simulink library "VSIGenLib"  (R2019b)
settings: Solver=VariableStepAuto  StartTime=0.0  StopTime=10.0  RelTol=1e-3
PostLoadFcn:
  | , if any(exist('dsrtsu_mdlpostloadfcn', 'file') ~= 0), dsrtsu_mdlpostloadfcn('Execute', bdroot); end,
undefined symbols (not defined in the file or in its folder): LIDAR, Ts_hil
libraries: simulink x76, $bdroot x46, etargetslib x30, ASCGenLib x26, dsmpblib x6
(part 2 of 3)

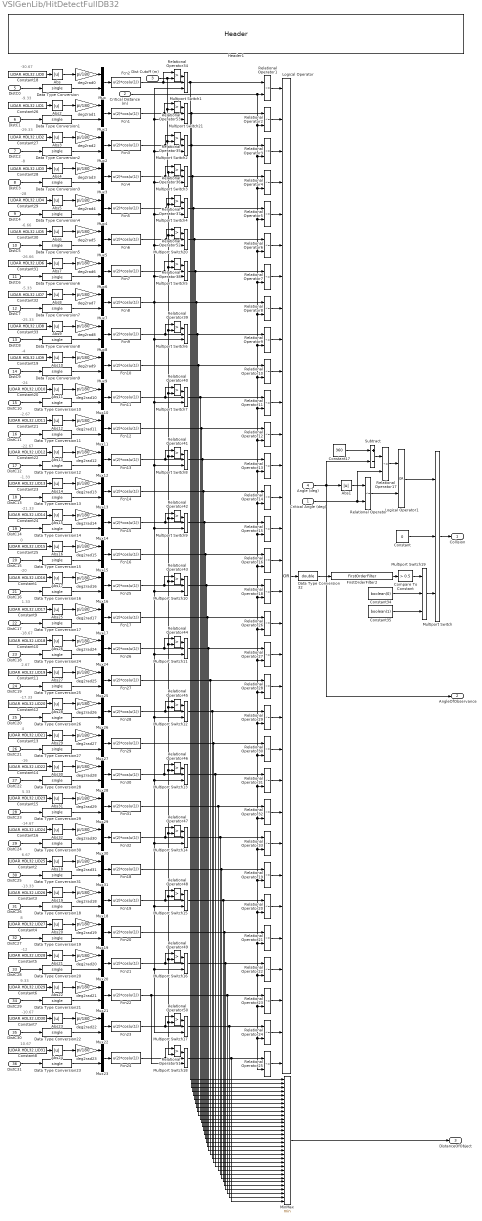
== system VSIGenLib/HitDetectFullDB32 ==
  note: -30.67
  note: -9.33
  note: -29.33
  note: -8
  note: -28
  note: -6.66
  note: -26.66
  note: -5.33
  note: -25.33
  note: -4
  note: -24
  note: -2.67
  note: 0
  note: -21.33
  note: -1.33
  note: -22.67
  note: -20
  note: 1.33
  note: -18.67
  note: 2.67
  note: -17.33
  note: 4
  note: -16
  note: 5.33
  note: -14.67
  note: 6.67
  note: -13.33
  note: 8
  note: 10.67
  note: -10.67
  note: 9.33
  note: -12
  Critical Angle (deg) : Inport
  Critical Distance (m) : Inport  Port=2
  Dist Cutoff (m) : Inport  Port=3
  Angle (deg) : Inport  Port=4
  DistC0 : Inport  Port=5
  DistC1 : Inport  Port=6
  DistC2 : Inport  Port=7
  DistC3 : Inport  Port=8
  DistC4 : Inport  Port=9
  DistC5 : Inport  Port=10
  DistC6 : Inport  Port=11
  DistC7 : Inport  Port=12
  DistC8 : Inport  Port=13
  DistC9 : Inport  Port=14
  DistC10 : Inport  Port=15
  DistC11 : Inport  Port=16
  DistC12 : Inport  Port=17
  DistC13 : Inport  Port=18
  DistC14 : Inport  Port=19
  DistC15 : Inport  Port=20
  DistC16 : Inport  Port=21
  DistC17 : Inport  Port=22
  DistC18 : Inport  Port=23
  DistC19 : Inport  Port=24
  DistC20 : Inport  Port=25
  DistC21 : Inport  Port=26
  DistC22 : Inport  Port=27
  DistC23 : Inport  Port=28
  DistC24 : Inport  Port=29
  DistC25 : Inport  Port=30
  DistC26 : Inport  Port=31
  DistC27 : Inport  Port=32
  DistC28 : Inport  Port=33
  DistC29 : Inport  Port=34
  DistC30 : Inport  Port=35
  DistC31 : Inport  Port=36
  Abs{,1..32} (33 alike) : Abs
  Compare To Constant : simulink/Logic and Bit Operations/Compare To Constant  relop=>  const=0.5  OutDataTypeStr=boolean
  Constant : Constant  Value=0
  Constant1 : Constant  Value=LIDAR.HDL32.LID16
  Constant10 : Constant  Value=LIDAR.HDL32.LID18
  Constant11 : Constant  Value=LIDAR.HDL32.LID19
  Constant12 : Constant  Value=LIDAR.HDL32.LID20
  Constant13 : Constant  Value=LIDAR.HDL32.LID21
  Constant14 : Constant  Value=LIDAR.HDL32.LID22
  Constant15 : Constant  Value=LIDAR.HDL32.LID23
  Constant16 : Constant  Value=LIDAR.HDL32.LID24
  Constant17 : Constant  Value=360
  Constant18 : Constant  Value=LIDAR.HDL32.LID0
  Constant19 : Constant  Value=LIDAR.HDL32.LID9
  Constant2 : Constant  Value=LIDAR.HDL32.LID25
  Constant20 : Constant  Value=LIDAR.HDL32.LID10
  Constant21 : Constant  Value=LIDAR.HDL32.LID11
  Constant22 : Constant  Value=LIDAR.HDL32.LID12
  Constant23 : Constant  Value=LIDAR.HDL32.LID13
  Constant24 : Constant  Value=LIDAR.HDL32.LID14
  Constant25 : Constant  Value=LIDAR.HDL32.LID15
  Constant26 : Constant  Value=LIDAR.HDL32.LID1
  Constant27 : Constant  Value=LIDAR.HDL32.LID2
  Constant28 : Constant  Value=LIDAR.HDL32.LID3
  Constant29 : Constant  Value=LIDAR.HDL32.LID4
  Constant3 : Constant  Value=LIDAR.HDL32.LID26
  Constant30 : Constant  Value=LIDAR.HDL32.LID5
  Constant31 : Constant  Value=LIDAR.HDL32.LID6
  Constant32 : Constant  Value=LIDAR.HDL32.LID7
  Constant33 : Constant  Value=LIDAR.HDL32.LID8
  Constant34 : Constant  Value=boolean(0)
  Constant35 : Constant  Value=boolean(1)
  Constant4 : Constant  Value=LIDAR.HDL32.LID27
  Constant5 : Constant  Value=LIDAR.HDL32.LID28
  Constant6 : Constant  Value=LIDAR.HDL32.LID29
  Constant7 : Constant  Value=LIDAR.HDL32.LID30
  Constant8 : Constant  Value=LIDAR.HDL32.LID31
  Constant9 : Constant  Value=LIDAR.HDL32.LID17
  Data Type Conversion{,1..31} (32 alike) : DataTypeConversion  OutDataTypeStr=single
  Data Type Conversion32 : DataTypeConversion  OutDataTypeStr=double
  Fcn{1..32} (32 alike) : Fcn  Expr=u(2)*cos(u(1))
  FirstOrderFilter2 : ASCGenLib/FirstOrderFilter  SystemSampleTime=-1
  Header1 : ASCGenLib/Header  not='L0 -30.67deg; L1 -9.33deg; L2 -29.33deg; L3 -8deg; L4 -28deg; L5 -6.66deg; L6 -26.66deg; L7 -5.33deg; L8 -25.33deg; L9 -4deg; L10 -24deg; L11 -2.67deg; L12 -22.67deg; L13 -1.33deg; L14 -21.33deg; L15 0deg\nL16 -20deg; L17 1.33deg; L18 -18.67deg; L19 2.67deg; L20 -17.33deg; L21 4deg; L22 -16deg; L23 5.33deg; L24 -14.67deg; L25 6.67deg; L26 -13.33deg; L27 8deg; L28 -12deg; L29 9.33deg; L30 -10.67deg; L31 10.67deg'
  Logical Operator : Logic  Operator=OR  Inputs=32  AllPortsSameDT=off  OutDataTypeStr=boolean
  Logical Operator1 : Logic  Operator=OR  AllPortsSameDT=off  OutDataTypeStr=boolean
  MinMax : MinMax  Inputs=32
  Multiport Switch{,1..21} (22 alike) : MultiPortSwitch  DataPortOrder=Zero-based contiguous  Inputs=2  zeroidx=on
  Mux{,1..31} (32 alike) : Mux  Inputs=2
  Relational Operator{,1..33} (34 alike) : RelationalOperator  Operator=<=  OutDataTypeStr=boolean  RndMeth=Simplest
  Relational Operator{34..53} (20 alike) : RelationalOperator  Operator=>  OutDataTypeStr=boolean  RndMeth=Simplest
  Subtract : Sum  Inputs=+-
  deg2rad{0..31} (32 alike) : Gain  Gain=pi/180  OutDataTypeStr=single
  Collision : Outport  VectorParamsAs1DForOutWhenUnconnected=off
  AngleOfObservance : Outport  Port=2  VectorParamsAs1DForOutWhenUnconnected=off
  DistanceOfObject : Outport  Port=3  VectorParamsAs1DForOutWhenUnconnected=off
  wires:
  Angle (deg)/1 -> Subtract/2, Abs1/1, AngleOfObservance/1
  Critical Angle (deg)/1 -> Relational Operator17/2, Relational Operator/2
  Relational Operator/1 -> Logical Operator1/2
  Constant/1 -> Multiport Switch/2
  Multiport Switch/1 -> Collision/1
  Relational Operator1/1 -> Logical Operator/1
  Constant18/1 -> Abs/1
  Mux/1 -> Fcn2/1
  Abs/1 -> deg2rad0/1
  Abs1/1 -> Relational Operator/1
  Constant26/1 -> Abs2/1
  Mux1/1 -> Fcn1/1
  Abs2/1 -> deg2rad1/1
  DistC0/1 -> Data Type Conversion/1
  DistC1/1 -> Data Type Conversion1/1
  Relational Operator2/1 -> Logical Operator/2
  Constant27/1 -> Abs3/1
  Mux2/1 -> Fcn3/1
  Abs3/1 -> deg2rad2/1
  Constant28/1 -> Abs4/1
  Mux3/1 -> Fcn4/1
  Abs4/1 -> deg2rad3/1
  DistC2/1 -> Data Type Conversion2/1
  DistC3/1 -> Data Type Conversion3/1
  Relational Operator3/1 -> Logical Operator/3
  Relational Operator4/1 -> Logical Operator/4
  Relational Operator5/1 -> Logical Operator/5
  Constant29/1 -> Abs5/1
  Abs5/1 -> deg2rad4/1
  Mux4/1 -> Fcn5/1
  deg2rad4/1 -> Mux4/1
  Constant30/1 -> Abs6/1
  Abs6/1 -> deg2rad5/1
  Mux5/1 -> Fcn6/1
  deg2rad5/1 -> Mux5/1
  DistC4/1 -> Data Type Conversion4/1
  DistC5/1 -> Data Type Conversion5/1
  Relational Operator6/1 -> Logical Operator/6
  Constant31/1 -> Abs7/1
  Abs7/1 -> deg2rad6/1
  Mux6/1 -> Fcn7/1
  deg2rad6/1 -> Mux6/1
  Constant32/1 -> Abs8/1
  Abs8/1 -> deg2rad7/1
  Mux7/1 -> Fcn8/1
  deg2rad7/1 -> Mux7/1
  DistC6/1 -> Data Type Conversion6/1
  DistC7/1 -> Data Type Conversion7/1
  Relational Operator7/1 -> Logical Operator/7
  Relational Operator8/1 -> Logical Operator/8
  Constant33/1 -> Abs9/1
  Abs9/1 -> deg2rad8/1
  Mux8/1 -> Fcn9/1
  deg2rad8/1 -> Mux8/1
  DistC8/1 -> Data Type Conversion8/1
  Relational Operator9/1 -> Logical Operator/9
  Relational Operator10/1 -> Logical Operator/10
  Constant19/1 -> Abs10/1
  Abs10/1 -> deg2rad9/1
  Mux9/1 -> Fcn10/1
  deg2rad9/1 -> Mux9/1
  Constant20/1 -> Abs11/1
  Abs11/1 -> deg2rad10/1
  Mux10/1 -> Fcn11/1
  deg2rad10/1 -> Mux10/1
  DistC9/1 -> Data Type Conversion9/1
  DistC10/1 -> Data Type Conversion10/1
  Relational Operator11/1 -> Logical Operator/11
  Constant21/1 -> Abs12/1
  Abs12/1 -> deg2rad11/1
  Mux11/1 -> Fcn12/1
  deg2rad11/1 -> Mux11/1
  Constant22/1 -> Abs13/1
  Abs13/1 -> deg2rad12/1
  Mux12/1 -> Fcn13/1
  deg2rad12/1 -> Mux12/1
  DistC11/1 -> Data Type Conversion11/1
  DistC12/1 -> Data Type Conversion12/1
  Relational Operator12/1 -> Logical Operator/12
  Relational Operator13/1 -> Logical Operator/13
  Constant23/1 -> Abs14/1
  Abs14/1 -> deg2rad13/1
  Mux13/1 -> Fcn14/1
  deg2rad13/1 -> Mux13/1
  Constant24/1 -> Abs15/1
  Abs15/1 -> deg2rad14/1
  Mux14/1 -> Fcn15/1
  deg2rad14/1 -> Mux14/1
  DistC13/1 -> Data Type Conversion13/1
  DistC14/1 -> Data Type Conversion14/1
  Relational Operator14/1 -> Logical Operator/14
  Relational Operator15/1 -> Logical Operator/15
  Constant25/1 -> Abs16/1
  Abs16/1 -> deg2rad15/1
  Mux15/1 -> Fcn16/1
  deg2rad15/1 -> Mux15/1
  DistC15/1 -> Data Type Conversion15/1
  Relational Operator16/1 -> Logical Operator/16
  Constant17/1 -> Subtract/1
  Subtract/1 -> Relational Operator17/1
  Logical Operator1/1 -> Multiport Switch/1
  Relational Operator17/1 -> Logical Operator1/1
  deg2rad0/1 -> Mux/1
  deg2rad1/1 -> Mux1/1
  deg2rad2/1 -> Mux2/1
  deg2rad3/1 -> Mux3/1
  MinMax/1 -> DistanceOfObject/1
  Data Type Conversion/1 -> Mux/2
  Data Type Conversion1/1 -> Mux1/2
  Data Type Conversion2/1 -> Mux2/2
  Data Type Conversion3/1 -> Mux3/2
  Data Type Conversion4/1 -> Mux4/2
  Data Type Conversion5/1 -> Mux5/2
  Data Type Conversion6/1 -> Mux6/2
  Data Type Conversion7/1 -> Mux7/2
  Data Type Conversion8/1 -> Mux8/2
  Data Type Conversion9/1 -> Mux9/2
  Data Type Conversion10/1 -> Mux10/2
  Data Type Conversion11/1 -> Mux11/2
  Data Type Conversion12/1 -> Mux12/2
  Data Type Conversion13/1 -> Mux13/2
  Data Type Conversion14/1 -> Mux14/2
  Data Type Conversion15/1 -> Mux15/2
  Constant1/1 -> Abs17/1
  Mux16/1 -> Fcn25/1
  Abs17/1 -> deg2rad16/1
  Constant9/1 -> Abs25/1
  Mux17/1 -> Fcn17/1
  Abs25/1 -> deg2rad17/1
  DistC16/1 -> Data Type Conversion16/1
  DistC17/1 -> Data Type Conversion17/1
  Constant10/1 -> Abs26/1
  Mux24/1 -> Fcn26/1
  Abs26/1 -> deg2rad24/1
  Constant11/1 -> Abs27/1
  Mux25/1 -> Fcn27/1
  Abs27/1 -> deg2rad25/1
  DistC18/1 -> Data Type Conversion24/1
  DistC19/1 -> Data Type Conversion25/1
  Constant12/1 -> Abs28/1
  Abs28/1 -> deg2rad26/1
  Mux26/1 -> Fcn28/1
  deg2rad26/1 -> Mux26/1
  Constant13/1 -> Abs29/1
  Abs29/1 -> deg2rad27/1
  Mux27/1 -> Fcn29/1
  deg2rad27/1 -> Mux27/1
  DistC20/1 -> Data Type Conversion26/1
  DistC21/1 -> Data Type Conversion27/1
  Constant14/1 -> Abs30/1
  Abs30/1 -> deg2rad28/1
  Mux28/1 -> Fcn30/1
  deg2rad28/1 -> Mux28/1
  Constant15/1 -> Abs31/1
  Abs31/1 -> deg2rad29/1
  Mux29/1 -> Fcn31/1
  deg2rad29/1 -> Mux29/1
  DistC22/1 -> Data Type Conversion28/1
  DistC23/1 -> Data Type Conversion29/1
  Constant16/1 -> Abs32/1
  Abs32/1 -> deg2rad30/1
  Mux30/1 -> Fcn32/1
  deg2rad30/1 -> Mux30/1
  DistC24/1 -> Data Type Conversion30/1
  Constant2/1 -> Abs18/1
  Abs18/1 -> deg2rad31/1
  Mux31/1 -> Fcn18/1
  deg2rad31/1 -> Mux31/1
  Constant3/1 -> Abs19/1
  Abs19/1 -> deg2rad18/1
  Mux18/1 -> Fcn19/1
  deg2rad18/1 -> Mux18/1
  DistC25/1 -> Data Type Conversion31/1
  DistC26/1 -> Data Type Conversion18/1
  Constant4/1 -> Abs20/1
  Abs20/1 -> deg2rad19/1
  Mux19/1 -> Fcn20/1
  deg2rad19/1 -> Mux19/1
  Constant5/1 -> Abs21/1
  Abs21/1 -> deg2rad20/1
  Mux20/1 -> Fcn21/1
  deg2rad20/1 -> Mux20/1
  DistC27/1 -> Data Type Conversion19/1
  DistC28/1 -> Data Type Conversion20/1
  Constant6/1 -> Abs22/1
  Abs22/1 -> deg2rad21/1
  Mux21/1 -> Fcn22/1
  deg2rad21/1 -> Mux21/1
  Constant7/1 -> Abs23/1
  Abs23/1 -> deg2rad22/1
  Mux22/1 -> Fcn23/1
  deg2rad22/1 -> Mux22/1
  DistC29/1 -> Data Type Conversion21/1
  DistC30/1 -> Data Type Conversion22/1
  Constant8/1 -> Abs24/1
  Abs24/1 -> deg2rad23/1
  Mux23/1 -> Fcn24/1
  deg2rad23/1 -> Mux23/1
  DistC31/1 -> Data Type Conversion23/1
  deg2rad16/1 -> Mux16/1
  deg2rad17/1 -> Mux17/1
  deg2rad24/1 -> Mux24/1
  deg2rad25/1 -> Mux25/1
  Data Type Conversion16/1 -> Mux16/2
  Data Type Conversion17/1 -> Mux17/2
  Data Type Conversion24/1 -> Mux24/2
  Data Type Conversion25/1 -> Mux25/2
  Data Type Conversion26/1 -> Mux26/2
  Data Type Conversion27/1 -> Mux27/2
  Data Type Conversion28/1 -> Mux28/2
  Data Type Conversion29/1 -> Mux29/2
  Data Type Conversion30/1 -> Mux30/2
  Data Type Conversion31/1 -> Mux31/2
  Data Type Conversion18/1 -> Mux18/2
  Data Type Conversion19/1 -> Mux19/2
  Data Type Conversion20/1 -> Mux20/2
  Data Type Conversion21/1 -> Mux21/2
  Data Type Conversion22/1 -> Mux22/2
  Data Type Conversion23/1 -> Mux23/2
  Relational Operator18/1 -> Logical Operator/17
  Relational Operator26/1 -> Logical Operator/18
  Relational Operator27/1 -> Logical Operator/19
  Relational Operator28/1 -> Logical Operator/20
  Relational Operator29/1 -> Logical Operator/21
  Relational Operator30/1 -> Logical Operator/22
  Relational Operator31/1 -> Logical Operator/23
  Relational Operator32/1 -> Logical Operator/24
  Relational Operator33/1 -> Logical Operator/25
  Relational Operator19/1 -> Logical Operator/26
  Relational Operator20/1 -> Logical Operator/27
  Relational Operator21/1 -> Logical Operator/28
  Relational Operator22/1 -> Logical Operator/29
  Relational Operator23/1 -> Logical Operator/30
  Relational Operator24/1 -> Logical Operator/31
  Relational Operator25/1 -> Logical Operator/32
  Critical Distance (m)/1 -> Relational Operator2/2, Relational Operator3/2, Relational Operator4/2, Relational Operator5/2, Relational Operator6/2, Relational Operator7/2, Relational Operator8/2, Relational Operator9/2, Relational Operator10/2, Relational Operator11/2, Relational Operator12/2, Relational Operator13/2, Relational Operator15/2, Relational Operator16/2, Relational Operator18/2, Relational Operator26/2, Relational Operator27/2, Relational Operator28/2, Relational Operator29/2, Relational Operator30/2, Relational Operator31/2, Relational Operator32/2, Relational Operator33/2, Relational Operator19/2, Relational Operator20/2, Relational Operator21/2, Relational Operator22/2, Relational Operator23/2, Relational Operator24/2, Relational Operator25/2, Relational Operator14/2, Relational Operator1/2
  Relational Operator34/1 -> Multiport Switch1/1
  Fcn2/1 -> Multiport Switch1/2, Relational Operator34/1
  Multiport Switch1/1 -> MinMax/1, Relational Operator1/1
  Relational Operator35/1 -> Multiport Switch2/1
  Multiport Switch2/1 -> MinMax/3, Relational Operator3/1
  Fcn3/1 -> Relational Operator35/1, Multiport Switch2/2
  Relational Operator36/1 -> Multiport Switch3/1
  Multiport Switch3/1 -> MinMax/4, Relational Operator4/1
  Fcn4/1 -> Multiport Switch3/2, Relational Operator36/1
  Relational Operator37/1 -> Multiport Switch4/1
  Fcn5/1 -> Relational Operator37/1, Multiport Switch4/2
  Multiport Switch4/1 -> MinMax/5, Relational Operator5/1
  Multiport Switch20/1 -> MinMax/6, Relational Operator6/1
  Relational Operator38/1 -> Multiport Switch5/1
  Multiport Switch5/1 -> MinMax/7, Relational Operator7/1
  Fcn7/1 -> Relational Operator38/1, Multiport Switch5/2
  Fcn8/1 -> MinMax/8, Relational Operator8/1, Multiport Switch6/3, Multiport Switch7/3, Multiport Switch10/3, Multiport Switch11/3, Multiport Switch12/3, Multiport Switch14/3, Multiport Switch15/3, Multiport Switch16/3, Multiport Switch17/3, Multiport Switch13/3, Multiport Switch9/3, Multiport Switch8/3, Multiport Switch5/3, Multiport Switch20/3, Multiport Switch4/3, Multiport Switch3/3, Multiport Switch21/3, Multiport Switch1/3, Multiport Switch2/3
  Relational Operator39/1 -> Multiport Switch6/1
  Fcn9/1 -> Relational Operator39/1, Multiport Switch6/2
  Multiport Switch6/1 -> MinMax/9, Relational Operator9/1
  Fcn10/1 -> MinMax/10, Relational Operator10/1
  Fcn11/1 -> Relational Operator40/1, Multiport Switch7/2
  Multiport Switch7/1 -> MinMax/11, Relational Operator11/1
  Fcn13/1 -> Relational Operator41/1, Multiport Switch8/2
  Multiport Switch8/1 -> MinMax/13, Relational Operator13/1
  Relational Operator40/1 -> Multiport Switch7/1
  Relational Operator41/1 -> Multiport Switch8/1
  Fcn14/1 -> MinMax/14, Relational Operator14/1
  Relational Operator42/1 -> Multiport Switch9/1
  Multiport Switch9/1 -> MinMax/15, Relational Operator15/1
  Fcn15/1 -> Relational Operator42/1, Multiport Switch9/2
  Fcn16/1 -> MinMax/16, Relational Operator16/1
  Relational Operator43/1 -> Multiport Switch10/1
  Fcn25/1 -> Relational Operator43/1, Multiport Switch10/2
  Multiport Switch10/1 -> MinMax/17, Relational Operator18/1
  Relational Operator44/1 -> Multiport Switch11/1
  Multiport Switch11/1 -> MinMax/19, Relational Operator27/1
  Fcn26/1 -> Relational Operator44/1, Multiport Switch11/2
  Fcn17/1 -> MinMax/18, Relational Operator26/1
  Fcn27/1 -> MinMax/20, Relational Operator28/1
  Relational Operator45/1 -> Multiport Switch12/1
  Multiport Switch12/1 -> MinMax/21, Relational Operator29/1
  Fcn28/1 -> Relational Operator45/1, Multiport Switch12/2
  Fcn29/1 -> MinMax/22, Relational Operator30/1
  Relational Operator46/1 -> Multiport Switch13/1
  Multiport Switch13/1 -> MinMax/23, Relational Operator31/1
  Fcn30/1 -> Relational Operator46/1, Multiport Switch13/2
  Relational Operator47/1 -> Multiport Switch14/1
  Multiport Switch14/1 -> MinMax/25, Relational Operator33/1
  Fcn32/1 -> Relational Operator47/1, Multiport Switch14/2
  Fcn31/1 -> MinMax/24, Relational Operator32/1
  Fcn18/1 -> MinMax/26, Relational Operator19/1
  Relational Operator48/1 -> Multiport Switch15/1
  Multiport Switch15/1 -> MinMax/27, Relational Operator20/1
  Fcn19/1 -> Relational Operator48/1, Multiport Switch15/2
  Fcn20/1 -> MinMax/28, Relational Operator21/1
  Relational Operator49/1 -> Multiport Switch16/1
  Multiport Switch16/1 -> MinMax/29, Relational Operator22/1
  Fcn21/1 -> Relational Operator49/1, Multiport Switch16/2
  Relational Operator50/1 -> Multiport Switch17/1
  Multiport Switch17/1 -> MinMax/31, Relational Operator24/1
  Fcn23/1 -> Relational Operator50/1, Multiport Switch17/2
  Fcn12/1 -> MinMax/12, Relational Operator12/1
  Fcn22/1 -> Multiport Switch18/3, MinMax/30, Relational Operator23/1
  Relational Operator51/1 -> Multiport Switch18/1
  Multiport Switch18/1 -> MinMax/32, Relational Operator25/1
  Fcn24/1 -> Relational Operator51/1, Multiport Switch18/2
  FirstOrderFilter2/1 -> Compare To Constant/1
  Constant34/1 -> Multiport Switch19/2
  Constant35/1 -> Multiport Switch19/3
  Compare To Constant/1 -> Multiport Switch19/1
  Multiport Switch19/1 -> Multiport Switch/3
  Data Type Conversion32/1 -> FirstOrderFilter2/1
  Logical Operator/1 -> Data Type Conversion32/1
  Relational Operator52/1 -> Multiport Switch20/1
  Fcn6/1 -> Relational Operator52/1, Multiport Switch20/2
  Fcn1/1 -> Relational Operator53/1, Multiport Switch21/2
  Relational Operator53/1 -> Multiport Switch21/1
  Dist Cutoff (m)/1 -> Relational Operator53/2, Relational Operator52/2, Relational Operator47/2, Relational Operator48/2, Relational Operator49/2, Relational Operator51/2, Relational Operator50/2, Relational Operator46/2, Relational Operator45/2, Relational Operator44/2, Relational Operator43/2, Relational Operator42/2, Relational Operator41/2, Relational Operator40/2, Relational Operator39/2, Relational Operator38/2, Relational Operator37/2, Relational Operator36/2, Relational Operator35/2, Relational Operator34/2
  Multiport Switch21/1 -> MinMax/2, Relational Operator2/1

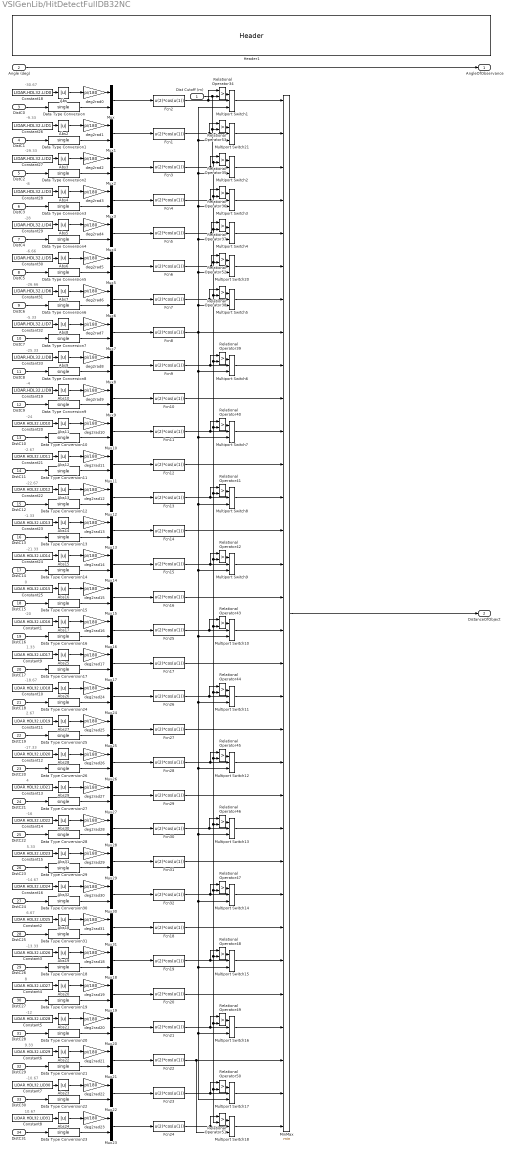
== system VSIGenLib/HitDetectFullDB32NC ==
  note: -30.67
  note: -9.33
  note: -8
  note: -6.66
  note: -26.66
  note: -5.33
  note: -4
  note: -24
  note: -2.67
  note: 0
  note: -1.33
  note: -22.67
  note: -29.33
  note: -20
  note: 1.33
  note: -28
  note: -18.67
  note: 2.67
  note: -17.33
  note: 4
  note: -25.33
  note: -16
  note: -14.67
  note: -13.33
  note: -21.33
  note: 8
  note: 10.67
  note: -10.67
  note: 9.33
  note: 5.33
  note: -12
  note: 6.67
  Dist Cutoff (m) : Inport
  Angle (deg) : Inport  Port=2
  DistC0 : Inport  Port=3
  DistC1 : Inport  Port=4
  DistC2 : Inport  Port=5
  DistC3 : Inport  Port=6
  DistC4 : Inport  Port=7
  DistC5 : Inport  Port=8
  DistC6 : Inport  Port=9
  DistC7 : Inport  Port=10
  DistC8 : Inport  Port=11
  DistC9 : Inport  Port=12
  DistC10 : Inport  Port=13
  DistC11 : Inport  Port=14
  DistC12 : Inport  Port=15
  DistC13 : Inport  Port=16
  DistC14 : Inport  Port=17
  DistC15 : Inport  Port=18
  DistC16 : Inport  Port=19
  DistC17 : Inport  Port=20
  DistC18 : Inport  Port=21
  DistC19 : Inport  Port=22
  DistC20 : Inport  Port=23
  DistC21 : Inport  Port=24
  DistC22 : Inport  Port=25
  DistC23 : Inport  Port=26
  DistC24 : Inport  Port=27
  DistC25 : Inport  Port=28
  DistC26 : Inport  Port=29
  DistC27 : Inport  Port=30
  DistC28 : Inport  Port=31
  DistC29 : Inport  Port=32
  DistC30 : Inport  Port=33
  DistC31 : Inport  Port=34
  Abs{,2..32} (32 alike) : Abs
  Constant1 : Constant  Value=LIDAR.HDL32.LID16
  Constant10 : Constant  Value=LIDAR.HDL32.LID18
  Constant11 : Constant  Value=LIDAR.HDL32.LID19
  Constant12 : Constant  Value=LIDAR.HDL32.LID20
  Constant13 : Constant  Value=LIDAR.HDL32.LID21
  Constant14 : Constant  Value=LIDAR.HDL32.LID22
  Constant15 : Constant  Value=LIDAR.HDL32.LID23
  Constant16 : Constant  Value=LIDAR.HDL32.LID24
  Constant18 : Constant  Value=LIDAR.HDL32.LID0
  Constant19 : Constant  Value=LIDAR.HDL32.LID9
  Constant2 : Constant  Value=LIDAR.HDL32.LID25
  Constant20 : Constant  Value=LIDAR.HDL32.LID10
  Constant21 : Constant  Value=LIDAR.HDL32.LID11
  Constant22 : Constant  Value=LIDAR.HDL32.LID12
  Constant23 : Constant  Value=LIDAR.HDL32.LID13
  Constant24 : Constant  Value=LIDAR.HDL32.LID14
  Constant25 : Constant  Value=LIDAR.HDL32.LID15
  Constant26 : Constant  Value=LIDAR.HDL32.LID1
  Constant27 : Constant  Value=LIDAR.HDL32.LID2
  Constant28 : Constant  Value=LIDAR.HDL32.LID3
  Constant29 : Constant  Value=LIDAR.HDL32.LID4
  Constant3 : Constant  Value=LIDAR.HDL32.LID26
  Constant30 : Constant  Value=LIDAR.HDL32.LID5
  Constant31 : Constant  Value=LIDAR.HDL32.LID6
  Constant32 : Constant  Value=LIDAR.HDL32.LID7
  Constant33 : Constant  Value=LIDAR.HDL32.LID8
  Constant4 : Constant  Value=LIDAR.HDL32.LID27
  Constant5 : Constant  Value=LIDAR.HDL32.LID28
  Constant6 : Constant  Value=LIDAR.HDL32.LID29
  Constant7 : Constant  Value=LIDAR.HDL32.LID30
  Constant8 : Constant  Value=LIDAR.HDL32.LID31
  Constant9 : Constant  Value=LIDAR.HDL32.LID17
  Data Type Conversion{,1..31} (32 alike) : DataTypeConversion  OutDataTypeStr=single
  Fcn{1..32} (32 alike) : Fcn  Expr=u(2)*cos(u(1))
  Header1 : ASCGenLib/Header  not='L0 -30.67deg; L1 -9.33deg; L2 -29.33deg; L3 -8deg; L4 -28deg; L5 -6.66deg; L6 -26.66deg; L7 -5.33deg; L8 -25.33deg; L9 -4deg; L10 -24deg; L11 -2.67deg; L12 -22.67deg; L13 -1.33deg; L14 -21.33deg; L15 0deg\nL16 -20deg; L17 1.33deg; L18 -18.67deg; L19 2.67deg; L20 -17.33deg; L21 4deg; L22 -16deg; L23 5.33deg; L24 -14.67deg; L25 6.67deg; L26 -13.33deg; L27 8deg; L28 -12deg; L29 9.33deg; L30 -10.67deg; L31 10.67deg'
  MinMax : MinMax  Inputs=32
  Multiport Switch{1..18,20..21} (20 alike) : MultiPortSwitch  DataPortOrder=Zero-based contiguous  Inputs=2  zeroidx=on
  Mux{,1..31} (32 alike) : Mux  Inputs=2
  Relational Operator{34..53} (20 alike) : RelationalOperator  Operator=>  OutDataTypeStr=boolean  RndMeth=Simplest
  deg2rad{0..31} (32 alike) : Gain  Gain=pi/180  OutDataTypeStr=single
  AngleOfObservance : Outport  VectorParamsAs1DForOutWhenUnconnected=off
  DistanceOfObject : Outport  Port=2  VectorParamsAs1DForOutWhenUnconnected=off
  wires:
  Multiport Switch16/1 -> MinMax/29
  Mux14/1 -> Fcn15/1
  Multiport Switch18/1 -> MinMax/32
  Mux17/1 -> Fcn17/1
  Abs6/1 -> deg2rad5/1
  Constant6/1 -> Abs22/1
  DistC3/1 -> Data Type Conversion3/1
  Relational Operator46/1 -> Multiport Switch13/1
  Dist Cutoff (m)/1 -> Relational Operator53/2, Relational Operator52/2, Relational Operator47/2, Relational Operator48/2, Relational Operator49/2, Relational Operator51/2, Relational Operator50/2, Relational Operator46/2, Relational Operator45/2, Relational Operator44/2, Relational Operator43/2, Relational Operator42/2, Relational Operator41/2, Relational Operator40/2, Relational Operator39/2, Relational Operator38/2, Relational Operator37/2, Relational Operator36/2, Relational Operator35/2, Relational Operator34/2
  deg2rad23/1 -> Mux23/1
  Multiport Switch14/1 -> MinMax/25
  Fcn2/1 -> Multiport Switch1/2, Relational Operator34/1
  Relational Operator40/1 -> Multiport Switch7/1
  Data Type Conversion/1 -> Mux/2
  DistC9/1 -> Data Type Conversion9/1
  DistC24/1 -> Data Type Conversion30/1
  Mux9/1 -> Fcn10/1
  deg2rad19/1 -> Mux19/1
  DistC5/1 -> Data Type Conversion5/1
  DistC0/1 -> Data Type Conversion/1
  Multiport Switch17/1 -> MinMax/31
  DistC25/1 -> Data Type Conversion31/1
  Fcn6/1 -> Relational Operator52/1, Multiport Switch20/2
  Abs24/1 -> deg2rad23/1
  Constant27/1 -> Abs3/1
  Constant8/1 -> Abs24/1
  Fcn21/1 -> Relational Operator49/1, Multiport Switch16/2
  Abs31/1 -> deg2rad29/1
  Multiport Switch8/1 -> MinMax/13
  DistC10/1 -> Data Type Conversion10/1
  deg2rad11/1 -> Mux11/1
  Relational Operator49/1 -> Multiport Switch16/1
  DistC27/1 -> Data Type Conversion19/1
  Abs15/1 -> deg2rad14/1
  Multiport Switch13/1 -> MinMax/23
  Relational Operator41/1 -> Multiport Switch8/1
  Fcn16/1 -> MinMax/16
  Fcn1/1 -> Relational Operator53/1, Multiport Switch21/2
  Fcn19/1 -> Relational Operator48/1, Multiport Switch15/2
  Data Type Conversion21/1 -> Mux21/2
  Fcn27/1 -> MinMax/20
  Fcn30/1 -> Relational Operator46/1, Multiport Switch13/2
  Multiport Switch20/1 -> MinMax/6
  Relational Operator39/1 -> Multiport Switch6/1
  DistC8/1 -> Data Type Conversion8/1
  Abs25/1 -> deg2rad17/1
  Mux20/1 -> Fcn21/1
  Abs/1 -> deg2rad0/1
  Data Type Conversion24/1 -> Mux24/2
  deg2rad12/1 -> Mux12/1
  Constant5/1 -> Abs21/1
  Fcn26/1 -> Relational Operator44/1, Multiport Switch11/2
  Fcn20/1 -> MinMax/28
  Relational Operator53/1 -> Multiport Switch21/1
  Fcn24/1 -> Relational Operator51/1, Multiport Switch18/2
  Fcn13/1 -> Relational Operator41/1, Multiport Switch8/2
  Fcn23/1 -> Relational Operator50/1, Multiport Switch17/2
  Relational Operator43/1 -> Multiport Switch10/1
  deg2rad16/1 -> Mux16/1
  Abs10/1 -> deg2rad9/1
  Relational Operator50/1 -> Multiport Switch17/1
  Abs22/1 -> deg2rad21/1
  deg2rad18/1 -> Mux18/1
  Multiport Switch9/1 -> MinMax/15
  Multiport Switch3/1 -> MinMax/4
  Mux23/1 -> Fcn24/1
  Fcn14/1 -> MinMax/14
  DistC11/1 -> Data Type Conversion11/1
  Constant13/1 -> Abs29/1
  Fcn10/1 -> MinMax/10
  Relational Operator38/1 -> Multiport Switch5/1
  Data Type Conversion1/1 -> Mux1/2
  Fcn9/1 -> Relational Operator39/1, Multiport Switch6/2
  Fcn8/1 -> MinMax/8, Multiport Switch6/3, Multiport Switch7/3, Multiport Switch10/3, Multiport Switch11/3, Multiport Switch12/3, Multiport Switch14/3, Multiport Switch15/3, Multiport Switch16/3, Multiport Switch17/3, Multiport Switch13/3, Multiport Switch9/3, Multiport Switch8/3, Multiport Switch5/3, Multiport Switch20/3, Multiport Switch4/3, Multiport Switch3/3, Multiport Switch21/3, Multiport Switch1/3, Multiport Switch2/3
  Constant9/1 -> Abs25/1
  Fcn12/1 -> MinMax/12
  Relational Operator48/1 -> Multiport Switch15/1
  Relational Operator52/1 -> Multiport Switch20/1
  Fcn28/1 -> Relational Operator45/1, Multiport Switch12/2
  Relational Operator37/1 -> Multiport Switch4/1
  deg2rad10/1 -> Mux10/1
  DistC26/1 -> Data Type Conversion18/1
  Multiport Switch10/1 -> MinMax/17
  deg2rad3/1 -> Mux3/1
  Multiport Switch5/1 -> MinMax/7
  Relational Operator44/1 -> Multiport Switch11/1
  Multiport Switch4/1 -> MinMax/5
  Fcn17/1 -> MinMax/18
  Fcn32/1 -> Relational Operator47/1, Multiport Switch14/2
  Fcn4/1 -> Multiport Switch3/2, Relational Operator36/1
  Relational Operator34/1 -> Multiport Switch1/1
  Abs23/1 -> deg2rad22/1
  Relational Operator36/1 -> Multiport Switch3/1
  Fcn3/1 -> Relational Operator35/1, Multiport Switch2/2
  Relational Operator35/1 -> Multiport Switch2/1
  deg2rad0/1 -> Mux/1
  Multiport Switch1/1 -> MinMax/1
  Data Type Conversion29/1 -> Mux29/2
  Data Type Conversion9/1 -> Mux9/2
  Data Type Conversion7/1 -> Mux7/2
  Fcn5/1 -> Relational Operator37/1, Multiport Switch4/2
  Constant3/1 -> Abs19/1
  deg2rad22/1 -> Mux22/1
  Abs32/1 -> deg2rad30/1
  DistC12/1 -> Data Type Conversion12/1
  Data Type Conversion26/1 -> Mux26/2
  Constant23/1 -> Abs14/1
  Data Type Conversion22/1 -> Mux22/2
  Mux27/1 -> Fcn29/1
  Data Type Conversion20/1 -> Mux20/2
  Data Type Conversion19/1 -> Mux19/2
  Mux19/1 -> Fcn20/1
  Data Type Conversion30/1 -> Mux30/2
  Data Type Conversion28/1 -> Mux28/2
  Data Type Conversion27/1 -> Mux27/2
  Relational Operator47/1 -> Multiport Switch14/1
  DistC17/1 -> Data Type Conversion17/1
  Data Type Conversion6/1 -> Mux6/2
  Constant10/1 -> Abs26/1
  Data Type Conversion16/1 -> Mux16/2
  Abs9/1 -> deg2rad8/1
  Fcn25/1 -> Relational Operator43/1, Multiport Switch10/2
  deg2rad24/1 -> Mux24/1
  deg2rad17/1 -> Mux17/1
  DistC31/1 -> Data Type Conversion23/1
  DistC30/1 -> Data Type Conversion22/1
  Constant11/1 -> Abs27/1
  Mux21/1 -> Fcn22/1
  Constant16/1 -> Abs32/1
  DistC28/1 -> Data Type Conversion20/1
  deg2rad20/1 -> Mux20/1
  Data Type Conversion3/1 -> Mux3/2
  deg2rad21/1 -> Mux21/1
  Abs21/1 -> deg2rad20/1
  Abs20/1 -> deg2rad19/1
  Constant4/1 -> Abs20/1
  deg2rad2/1 -> Mux2/1
  Abs19/1 -> deg2rad18/1
  deg2rad14/1 -> Mux14/1
  Abs18/1 -> deg2rad31/1
  Mux31/1 -> Fcn18/1
  Constant2/1 -> Abs18/1
  Abs26/1 -> deg2rad24/1
  deg2rad30/1 -> Mux30/1
  Mux30/1 -> Fcn32/1
  Constant15/1 -> Abs31/1
  Data Type Conversion17/1 -> Mux17/2
  Abs14/1 -> deg2rad13/1
  Fcn15/1 -> Relational Operator42/1, Multiport Switch9/2
  DistC16/1 -> Data Type Conversion16/1
  Constant18/1 -> Abs/1
  DistC21/1 -> Data Type Conversion27/1
  DistC20/1 -> Data Type Conversion26/1
  Mux25/1 -> Fcn27/1
  deg2rad27/1 -> Mux27/1
  deg2rad26/1 -> Mux26/1
  Multiport Switch12/1 -> MinMax/21
  Mux26/1 -> Fcn28/1
  Abs28/1 -> deg2rad26/1
  Constant12/1 -> Abs28/1
  Multiport Switch21/1 -> MinMax/2
  Mux12/1 -> Fcn13/1
  Abs27/1 -> deg2rad25/1
  Mux24/1 -> Fcn26/1
  Relational Operator42/1 -> Multiport Switch9/1
  Fcn11/1 -> Relational Operator40/1, Multiport Switch7/2
  deg2rad9/1 -> Mux9/1
  Abs17/1 -> deg2rad16/1
  Constant7/1 -> Abs23/1
  Mux16/1 -> Fcn25/1
  Constant1/1 -> Abs17/1
  deg2rad29/1 -> Mux29/1
  Data Type Conversion15/1 -> Mux15/2
  Multiport Switch6/1 -> MinMax/9
  Mux/1 -> Fcn2/1
  Data Type Conversion14/1 -> Mux14/2
  Data Type Conversion13/1 -> Mux13/2
  Mux18/1 -> Fcn19/1
  Data Type Conversion12/1 -> Mux12/2
  Data Type Conversion10/1 -> Mux10/2
  Data Type Conversion23/1 -> Mux23/2
  Data Type Conversion8/1 -> Mux8/2
  Data Type Conversion25/1 -> Mux25/2
  Abs29/1 -> deg2rad27/1
  Data Type Conversion5/1 -> Mux5/2
  DistC22/1 -> Data Type Conversion28/1
  Fcn7/1 -> Relational Operator38/1, Multiport Switch5/2
  Multiport Switch2/1 -> MinMax/3
  Data Type Conversion4/1 -> Mux4/2
  Abs11/1 -> deg2rad10/1
  DistC13/1 -> Data Type Conversion13/1
  deg2rad31/1 -> Mux31/1
  Abs13/1 -> deg2rad12/1
  Abs12/1 -> deg2rad11/1
  Constant22/1 -> Abs13/1
  Constant20/1 -> Abs11/1
  Mux28/1 -> Fcn30/1
  Abs16/1 -> deg2rad15/1
  Relational Operator51/1 -> Multiport Switch18/1
  Constant19/1 -> Abs10/1
  Constant24/1 -> Abs15/1
  Multiport Switch15/1 -> MinMax/27
  deg2rad8/1 -> Mux8/1
  deg2rad15/1 -> Mux15/1
  Mux22/1 -> Fcn23/1
  Mux29/1 -> Fcn31/1
  Mux8/1 -> Fcn9/1
  Data Type Conversion18/1 -> Mux18/2
  Constant26/1 -> Abs2/1
  Fcn18/1 -> MinMax/26
  DistC6/1 -> Data Type Conversion6/1
  Abs8/1 -> deg2rad7/1
  DistC23/1 -> Data Type Conversion29/1
  Constant32/1 -> Abs8/1
  deg2rad1/1 -> Mux1/1
  Data Type Conversion11/1 -> Mux11/2
  deg2rad6/1 -> Mux6/1
  Fcn31/1 -> MinMax/24
  DistC14/1 -> Data Type Conversion14/1
  deg2rad25/1 -> Mux25/1
  Constant31/1 -> Abs7/1
  DistC4/1 -> Data Type Conversion4/1
  deg2rad5/1 -> Mux5/1
  Data Type Conversion2/1 -> Mux2/2
  Data Type Conversion31/1 -> Mux31/2
  Mux5/1 -> Fcn6/1
  Constant30/1 -> Abs6/1
  deg2rad28/1 -> Mux28/1
  deg2rad4/1 -> Mux4/1
  Fcn22/1 -> MinMax/30, Multiport Switch18/3
  Multiport Switch11/1 -> MinMax/19
  Abs5/1 -> deg2rad4/1
  DistC18/1 -> Data Type Conversion24/1
  Mux11/1 -> Fcn12/1
  DistC29/1 -> Data Type Conversion21/1
  Constant29/1 -> Abs5/1
  deg2rad13/1 -> Mux13/1
  DistC15/1 -> Data Type Conversion15/1
  DistC1/1 -> Data Type Conversion1/1
  Mux7/1 -> Fcn8/1
  Mux1/1 -> Fcn1/1
  deg2rad7/1 -> Mux7/1
  DistC7/1 -> Data Type Conversion7/1
  DistC19/1 -> Data Type Conversion25/1
  Constant25/1 -> Abs16/1
  Abs4/1 -> deg2rad3/1
  Constant28/1 -> Abs4/1
  Abs7/1 -> deg2rad6/1
  Abs3/1 -> deg2rad2/1
  Constant33/1 -> Abs9/1
  Abs30/1 -> deg2rad28/1
  Mux2/1 -> Fcn3/1
  Fcn29/1 -> MinMax/22
  Mux10/1 -> Fcn11/1
  Abs2/1 -> deg2rad1/1
  Mux13/1 -> Fcn14/1
  Mux15/1 -> Fcn16/1
  Mux4/1 -> Fcn5/1
  Angle (deg)/1 -> AngleOfObservance/1
  Constant21/1 -> Abs12/1
  Relational Operator45/1 -> Multiport Switch12/1
  Mux3/1 -> Fcn4/1
  Constant14/1 -> Abs30/1
  Mux6/1 -> Fcn7/1
  Multiport Switch7/1 -> MinMax/11
  DistC2/1 -> Data Type Conversion2/1
  MinMax/1 -> DistanceOfObject/1

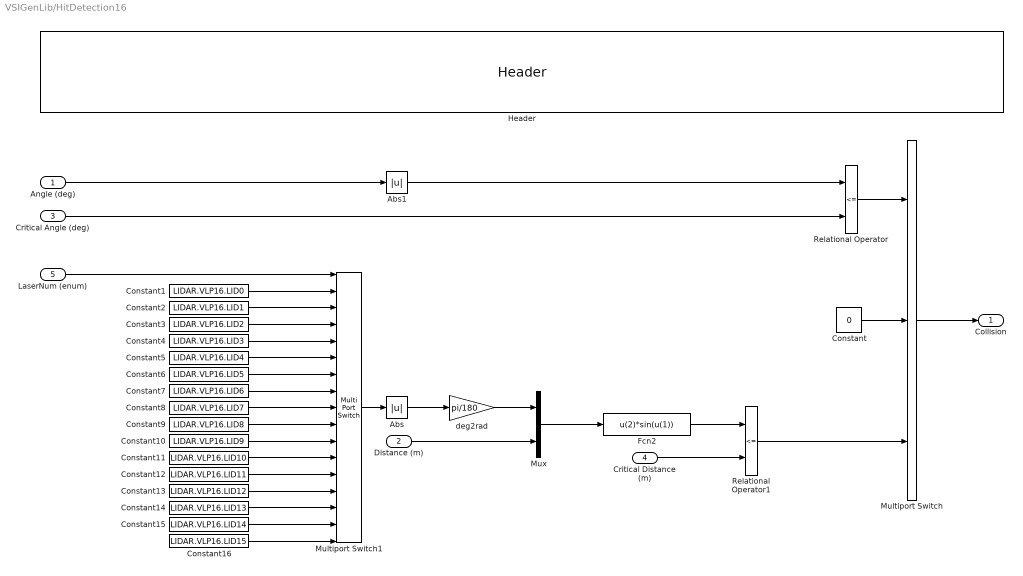
== system VSIGenLib/HitDetection16 ==
  Angle (deg) : Inport
  Distance (m) : Inport  Port=2
  Critical Angle (deg) : Inport  Port=3
  Critical Distance (m) : Inport  Port=4
  LaserNum (enum) : Inport  Port=5
  Abs : Abs
  Abs1 : Abs
  Constant : Constant  Value=0
  Constant1 : Constant  Value=LIDAR.VLP16.LID0
  Constant10 : Constant  Value=LIDAR.VLP16.LID9
  Constant11 : Constant  Value=LIDAR.VLP16.LID10
  Constant12 : Constant  Value=LIDAR.VLP16.LID11
  Constant13 : Constant  Value=LIDAR.VLP16.LID12
  Constant14 : Constant  Value=LIDAR.VLP16.LID13
  Constant15 : Constant  Value=LIDAR.VLP16.LID14
  Constant16 : Constant  Value=LIDAR.VLP16.LID15
  Constant2 : Constant  Value=LIDAR.VLP16.LID1
  Constant3 : Constant  Value=LIDAR.VLP16.LID2
  Constant4 : Constant  Value=LIDAR.VLP16.LID3
  Constant5 : Constant  Value=LIDAR.VLP16.LID4
  Constant6 : Constant  Value=LIDAR.VLP16.LID5
  Constant7 : Constant  Value=LIDAR.VLP16.LID6
  Constant8 : Constant  Value=LIDAR.VLP16.LID7
  Constant9 : Constant  Value=LIDAR.VLP16.LID8
  Fcn2 : Fcn  Expr=u(2)*sin(u(1))
  Header : $bdroot/Header  not=''
  Multiport Switch : MultiPortSwitch  DataPortOrder=Zero-based contiguous  Inputs=2  zeroidx=on
  Multiport Switch1 : MultiPortSwitch  DataPortOrder=Zero-based contiguous  Inputs=16  zeroidx=on
  Mux : Mux  Inputs=2
  Relational Operator : RelationalOperator  Operator=<=  OutDataTypeStr=boolean  RndMeth=Simplest
  Relational Operator1 : RelationalOperator  Operator=<=  OutDataTypeStr=boolean  RndMeth=Simplest
  deg2rad : Gain  Gain=pi/180
  Collision : Outport  VectorParamsAs1DForOutWhenUnconnected=off
  wires:
  Angle (deg)/1 -> Abs1/1
  Critical Angle (deg)/1 -> Relational Operator/2
  Distance (m)/1 -> Mux/2
  Critical Distance (m)/1 -> Relational Operator1/2
  Relational Operator/1 -> Multiport Switch/1
  Constant/1 -> Multiport Switch/2
  Multiport Switch/1 -> Collision/1
  Relational Operator1/1 -> Multiport Switch/3
  LaserNum (enum)/1 -> Multiport Switch1/1
  Constant1/1 -> Multiport Switch1/2
  Constant2/1 -> Multiport Switch1/3
  Constant9/1 -> Multiport Switch1/10
  Constant10/1 -> Multiport Switch1/11
  Constant7/1 -> Multiport Switch1/8
  Constant8/1 -> Multiport Switch1/9
  Constant3/1 -> Multiport Switch1/4
  Constant4/1 -> Multiport Switch1/5
  Constant15/1 -> Multiport Switch1/16
  Constant16/1 -> Multiport Switch1/17
  Constant5/1 -> Multiport Switch1/6
  Constant6/1 -> Multiport Switch1/7
  Constant13/1 -> Multiport Switch1/14
  Constant14/1 -> Multiport Switch1/15
  Constant11/1 -> Multiport Switch1/12
  Constant12/1 -> Multiport Switch1/13
  Multiport Switch1/1 -> Abs/1
  Abs/1 -> deg2rad/1
  Mux/1 -> Fcn2/1
  deg2rad/1 -> Mux/1
  Fcn2/1 -> Relational Operator1/1
  Abs1/1 -> Relational Operator/1

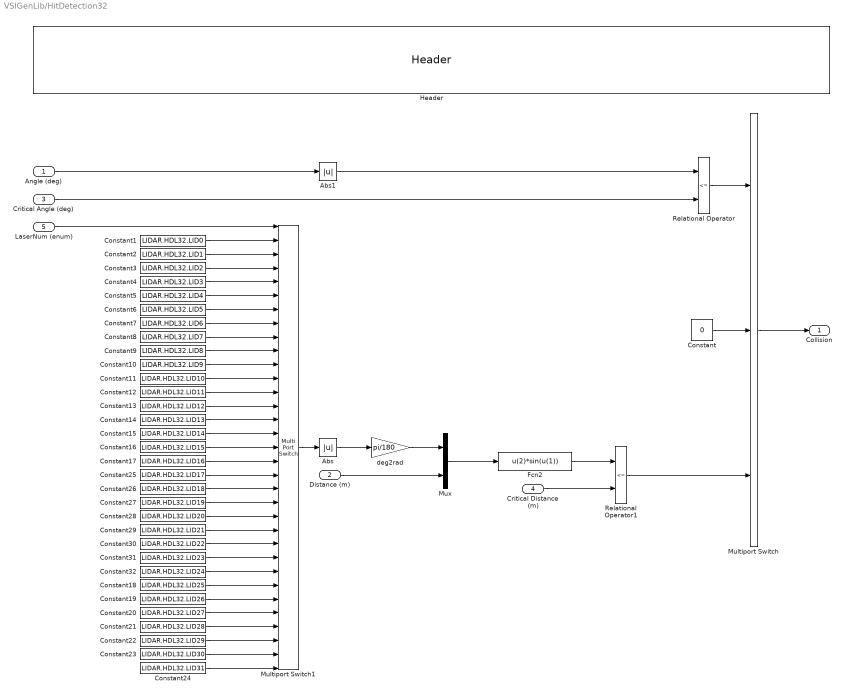
== system VSIGenLib/HitDetection32 ==
  Angle (deg) : Inport
  Distance (m) : Inport  Port=2
  Critical Angle (deg) : Inport  Port=3
  Critical Distance (m) : Inport  Port=4
  LaserNum (enum) : Inport  Port=5
  Abs : Abs
  Abs1 : Abs
  Constant : Constant  Value=0
  Constant1 : Constant  Value=LIDAR.HDL32.LID0
  Constant10 : Constant  Value=LIDAR.HDL32.LID9
  Constant11 : Constant  Value=LIDAR.HDL32.LID10
  Constant12 : Constant  Value=LIDAR.HDL32.LID11
  Constant13 : Constant  Value=LIDAR.HDL32.LID12
  Constant14 : Constant  Value=LIDAR.HDL32.LID13
  Constant15 : Constant  Value=LIDAR.HDL32.LID14
  Constant16 : Constant  Value=LIDAR.HDL32.LID15
  Constant17 : Constant  Value=LIDAR.HDL32.LID16
  Constant18 : Constant  Value=LIDAR.HDL32.LID25
  Constant19 : Constant  Value=LIDAR.HDL32.LID26
  Constant2 : Constant  Value=LIDAR.HDL32.LID1
  Constant20 : Constant  Value=LIDAR.HDL32.LID27
  Constant21 : Constant  Value=LIDAR.HDL32.LID28
  Constant22 : Constant  Value=LIDAR.HDL32.LID29
  Constant23 : Constant  Value=LIDAR.HDL32.LID30
  Constant24 : Constant  Value=LIDAR.HDL32.LID31
  Constant25 : Constant  Value=LIDAR.HDL32.LID17
  Constant26 : Constant  Value=LIDAR.HDL32.LID18
  Constant27 : Constant  Value=LIDAR.HDL32.LID19
  Constant28 : Constant  Value=LIDAR.HDL32.LID20
  Constant29 : Constant  Value=LIDAR.HDL32.LID21
  Constant3 : Constant  Value=LIDAR.HDL32.LID2
  Constant30 : Constant  Value=LIDAR.HDL32.LID22
  Constant31 : Constant  Value=LIDAR.HDL32.LID23
  Constant32 : Constant  Value=LIDAR.HDL32.LID24
  Constant4 : Constant  Value=LIDAR.HDL32.LID3
  Constant5 : Constant  Value=LIDAR.HDL32.LID4
  Constant6 : Constant  Value=LIDAR.HDL32.LID5
  Constant7 : Constant  Value=LIDAR.HDL32.LID6
  Constant8 : Constant  Value=LIDAR.HDL32.LID7
  Constant9 : Constant  Value=LIDAR.HDL32.LID8
  Fcn2 : Fcn  Expr=u(2)*sin(u(1))
  Header : ASCGenLib/Header  not=''
  Multiport Switch : MultiPortSwitch  DataPortOrder=Zero-based contiguous  Inputs=2  zeroidx=on
  Multiport Switch1 : MultiPortSwitch  DataPortOrder=Zero-based contiguous  Inputs=32  zeroidx=on
  Mux : Mux  Inputs=2
  Relational Operator : RelationalOperator  Operator=<=  OutDataTypeStr=boolean  RndMeth=Simplest
  Relational Operator1 : RelationalOperator  Operator=<=  OutDataTypeStr=boolean  RndMeth=Simplest
  deg2rad : Gain  Gain=pi/180
  Collision : Outport  VectorParamsAs1DForOutWhenUnconnected=off
  wires:
  Angle (deg)/1 -> Abs1/1
  Critical Angle (deg)/1 -> Relational Operator/2
  Distance (m)/1 -> Mux/2
  Critical Distance (m)/1 -> Relational Operator1/2
  Relational Operator/1 -> Multiport Switch/1
  Constant/1 -> Multiport Switch/2
  Multiport Switch/1 -> Collision/1
  Relational Operator1/1 -> Multiport Switch/3
  LaserNum (enum)/1 -> Multiport Switch1/1
  Constant1/1 -> Multiport Switch1/2
  Constant2/1 -> Multiport Switch1/3
  Constant9/1 -> Multiport Switch1/10
  Constant10/1 -> Multiport Switch1/11
  Constant7/1 -> Multiport Switch1/8
  Constant8/1 -> Multiport Switch1/9
  Constant3/1 -> Multiport Switch1/4
  Constant4/1 -> Multiport Switch1/5
  Constant15/1 -> Multiport Switch1/16
  Constant16/1 -> Multiport Switch1/17
  Constant5/1 -> Multiport Switch1/6
  Constant6/1 -> Multiport Switch1/7
  Constant13/1 -> Multiport Switch1/14
  Constant14/1 -> Multiport Switch1/15
  Constant11/1 -> Multiport Switch1/12
  Constant12/1 -> Multiport Switch1/13
  Multiport Switch1/1 -> Abs/1
  Abs/1 -> deg2rad/1
  Mux/1 -> Fcn2/1
  deg2rad/1 -> Mux/1
  Fcn2/1 -> Relational Operator1/1
  Abs1/1 -> Relational Operator/1
  Constant17/1 -> Multiport Switch1/18
  Constant18/1 -> Multiport Switch1/27
  Constant19/1 -> Multiport Switch1/28
  Constant20/1 -> Multiport Switch1/29
  Constant21/1 -> Multiport Switch1/30
  Constant22/1 -> Multiport Switch1/31
  Constant23/1 -> Multiport Switch1/32
  Constant24/1 -> Multiport Switch1/33
  Constant25/1 -> Multiport Switch1/19
  Constant26/1 -> Multiport Switch1/20
  Constant27/1 -> Multiport Switch1/21
  Constant28/1 -> Multiport Switch1/22
  Constant29/1 -> Multiport Switch1/23
  Constant30/1 -> Multiport Switch1/24
  Constant31/1 -> Multiport Switch1/25
  Constant32/1 -> Multiport Switch1/26

== system VSIGenLib/IHoldValue ==
  Data : Inport
  Header : $bdroot/Header  not=''
  HoldVal : Stateflow chart  TreatAsAtomicUnit=on
  Unit Delay : UnitDelay  SampleTime=-1  HasFrameUpgradeWarning=on
  "Data " : Outport  VectorParamsAs1DForOutWhenUnconnected=off
  wires:
  Data/1 -> HoldVal/1(In), Unit Delay/1
  HoldVal/1(Out) -> "Data "/1
  Unit Delay/1 -> HoldVal/2(DIn)
